simulink model "robot_prototype_simulation_test_v1"  (R2022b)
settings: Solver=FixedStepDiscrete  StartTime=0.0  StopTime=10.0  FixedStep=T_S  RelTol=1e-3  EnableMultiTasking=on
values from neighbouring files (symbols this model uses):
  T_S = 10e-3    (= 0.01)    [robot_prototype_init.m]
libraries: SignalEditorBlockLib x1
settings Model: ExtModeTrigDuration=2  Creator=hp  LastModifiedBy=hp
settings SolverCC: PositivePriorityOrder=on
settings OptimizationCC: EnhancedBackFolding=on  PassReuseOutputArgsAs=Individual arguments  ZeroExternalMemoryAtStartup=off  ZeroInternalMemoryAtStartup=off  MaxStackSize=64  OptimizeBlockOrder=speed  DifferentSizesBufferReuse=on  OptimizationCustomize=off  EfficientTunableParamExpr=on
settings DebuggingCC: ParameterTunabilityLossMsg=error
settings HardwareCC: ProdBitPerPointer=32  ProdBitPerSizeT=32  ProdBitPerPtrDiffT=32  ProdLargestAtomicInteger=Long  ProdWordSize=32  ProdHWDeviceType=ARM Compatible->ARM 9
settings SFSimCC: MATLABDynamicMemAlloc=off
settings RTWCC: Description=Embedded Coder  SystemTargetFile=ert.tlc  HardwareBoard=LEGO MINDSTORMS EV3  TLCOptions="-aInlineSetEventsForThisBaseRateFcn=TLC_FALSE -aSuppressMultiTaskScheduler=TLC_FALSE  -aRateBasedStepFcn=0"  TemplateMakefile=ert_default_tmf  Toolchain=Sourcery G++ Lite v2009q3
settings CodeAppCC: ForceParamTrailComments=on  IgnoreCustomStorageClasses=off  OperatorAnnotations=on  SimulinkDataObjDesc=on  SFDataObjDesc=on  InsertBlockDesc=on
settings ERTTargetCC: SupportContinuousTime=on  SupportVariableSizeSignals=on  ExtModeTransport=2  ExtModeStaticAlloc=on  ExtModeMexFile=ext_xcp  ExtModeIntrfLevel=Level2 - Open

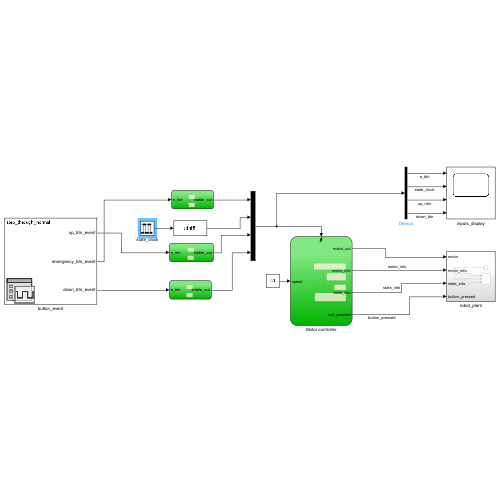
[thumbnail: Simulink's stored preview of the top-level diagram]
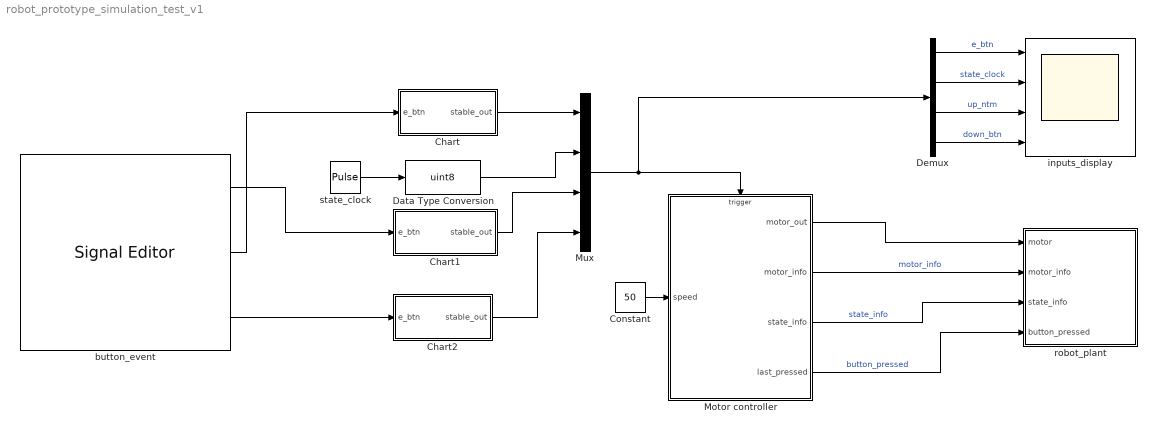
== system robot_prototype_simulation_test_v1 ==
  Chart : Stateflow chart  TreatAsAtomicUnit=on
  Chart1 : Stateflow chart  TreatAsAtomicUnit=on
  Chart2 : Stateflow chart  TreatAsAtomicUnit=on
  Constant : Constant  Value=50
  Data Type Conversion : DataTypeConversion  OutMin=0  OutMax=255  OutDataTypeStr=uint8  SaturateOnIntegerOverflow=off  RndMeth=Floor
  Demux : Demux
  Motor controller : Stateflow chart  TreatAsAtomicUnit=on
  Mux : Mux
  button_event : SignalEditorBlockLib/Signal Editor  FileName=step_through_signal_source.mat  ActiveScenario=step_through_normal  ActiveSignal=up_btn_event  IsBus=off  OutputBusObjectStr=Bus: BusObject  SampleTime=0  Interpolate=off  ZeroCross=off  OutputAfterFinalValue=Setting to zero  Unit=inherit  PreserveSignalName=on
  inputs_display : Scope  NumInputPorts=4
  robot_plant : Subsystem
  state_clock : DiscretePulseGenerator  Period=100  PulseWidth=50  PhaseDelay=20  SampleTime=T_S
  wires:
  button_event/2 -> Chart/1(e_btn)
  button_event/3 -> Chart2/1(e_btn)
  Constant/1 -> Motor controller/1(speed)
  button_event/1 -> Chart1/1(e_btn)
  Chart/1(stable_out) -> Mux/1
  state_clock/1 -> Data Type Conversion/1
  Mux/1 -> Demux/1, Motor controller/Trigger
  Data Type Conversion/1 -> Mux/2
  Chart1/1(stable_out) -> Mux/3
  Chart2/1(stable_out) -> Mux/4
  Motor controller/1(motor_out) -> robot_plant/1(motor)
  Motor controller/2(motor_info) -> robot_plant/2(motor_info)  "motor_info"
  Motor controller/3(state_info) -> robot_plant/3(state_info)  "state_info"
  Motor controller/4(last_pressed) -> robot_plant/4(button_pressed)  "button_pressed"
  Demux/1 -> inputs_display/1  "e_btn"
  Demux/3 -> inputs_display/3  "up_ntm"
  Demux/2 -> inputs_display/2  "state_clock"
  Demux/4 -> inputs_display/4  "down_btn"

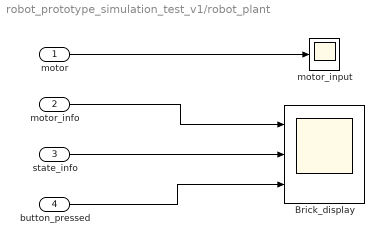
== system robot_prototype_simulation_test_v1/robot_plant ==
  motor : Inport
  motor_info : Inport  Port=2
  state_info : Inport  Port=3
  button_pressed : Inport  Port=4
  Brick_display : Scope  NumInputPorts=3
  motor_input : Scope
  wires:
  motor_info/1 -> Brick_display/1
  motor/1 -> motor_input/1
  state_info/1 -> Brick_display/2
  button_pressed/1 -> Brick_display/3

== stateflow chart robot_prototype_simulation_test_v1/Chart ==
  state off
    entry:
    stable_out = 0
  note: ]
  state on
    entry:
    stable_out = 1
  (default) -> off
  on -> off : [duration(e_btn<0.3) > 20e-3]
  off -> on : [duration(e_btn> 0.7) > 20e-3]
  data: e_btn input; stable_out output uint8

== stateflow chart robot_prototype_simulation_test_v1/Motor controller ==
  note: button_type is internal variable used to store which button was pressed
      | 0 = no button press
      | 1 = down
      | 2 = up
      | 3 = emergency_button
  state state_off
    entry:
    motor_out = 0;
    motor_info = 0;
    state_info = 0;
    last_pressed = button_type;
    e_press_count = 0;
  state emergency_stop
    entry:
    motor_out = 0;
    motor_info = 0;
    state_info = 2;
    last_pressed = button_type;
  state intermediate
    entry:
    e_press_count = e_press_count+1;
  state go
    entry:
    motor_out = speed;
    motor_info = 1;
    state_info = 1;
    last_pressed = button_type;
    e_press_count = 0;
  (default) -> state_off
  go -> state_off [order 2] : down_btn{button_type = 1}
  state_off -> go : up_btn{button_type = 2}
  go -> emergency_stop [order 1] : emergency_btn{button_type = 3}
  emergency_stop -> go [order 2] : [e_press_count == 2]
  emergency_stop -> intermediate [order 1] : emergency_btn
  intermediate -> emergency_stop [order 1] : after(0.5, sec){e_press_count = 0}
  intermediate -> emergency_stop [order 2] : emergency_btn{e_press_count = e_press_count+1}
  data: motor_out output; speed input; motor_info output; state_info output; button_type local =0; last_pressed output; e_press_count local =0
  events: emergency_btn input RISING_EDGE_EVENT; active_chart input RISING_EDGE_EVENT; up_btn input RISING_EDGE_EVENT; down_btn input RISING_EDGE_EVENT

== stateflow chart robot_prototype_simulation_test_v1/Chart1 ==
  state off
    entry:
    stable_out = 0
  note: ]
  state on
    entry:
    stable_out = 1
  (default) -> off
  on -> off : [duration(e_btn<0.3) > 20e-3]
  off -> on : [duration(e_btn> 0.7) > 20e-3]
  data: e_btn input; stable_out output uint8

== stateflow chart robot_prototype_simulation_test_v1/Chart2 ==
  state off
    entry:
    stable_out = 0
  note: ]
  state on
    entry:
    stable_out = 1
  (default) -> off
  on -> off : [duration(e_btn<0.3) > 20e-3]
  off -> on : [duration(e_btn> 0.7) > 20e-3]
  data: e_btn input; stable_out output uint8
